simulink model "vehicle_dynamic"  (R2022b)
settings: Solver=VariableStepAuto  StartTime=0.0  StopTime=30  RelTol=1e-3
values from neighbouring files (symbols this model uses):
  vx = 14    [vehicle_lateral_control_LMIs_3states_auto.m]
undefined symbols (not defined in the file or in its folder): K_gain_lin
settings Model: Creator=phatdo  LastModifiedBy=phatdo
settings DataIOCC: ReturnWorkspaceOutputs=off

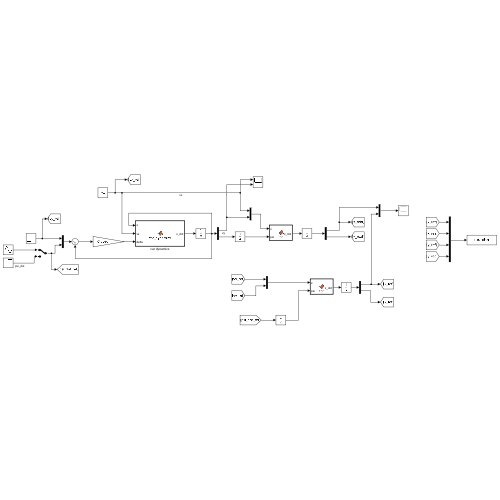
[thumbnail: Simulink's stored preview of the top-level diagram]
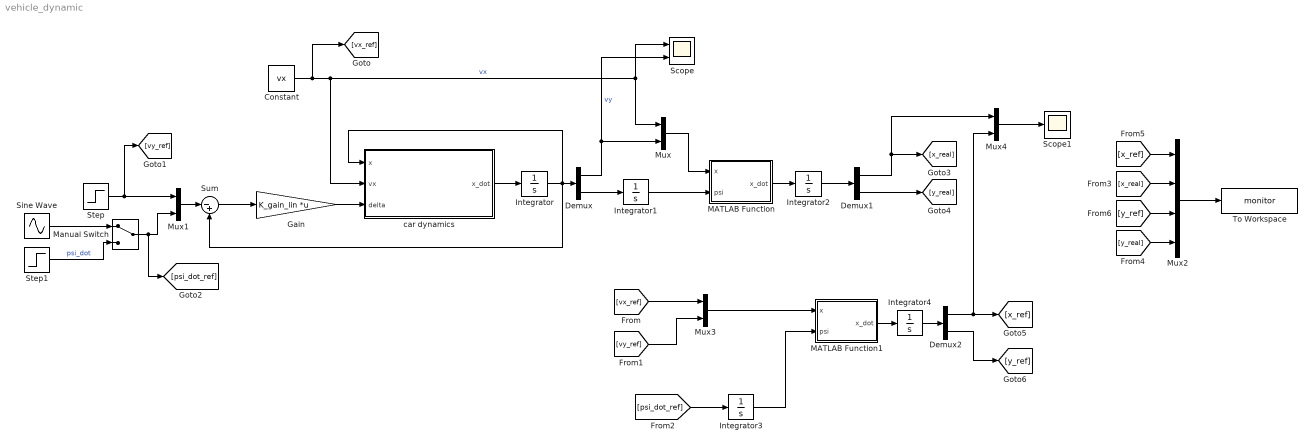
== system vehicle_dynamic ==
  Constant : Constant  Value=vx
  Demux : Demux  Outputs=2
  Demux1 : Demux  Outputs=2
  Demux2 : Demux  Outputs=2
  Gain : Gain  Gain=K_gain_lin  Multiplication=Matrix(K*u) (u vector)
  Integrator{,1..4} (5 alike) : Integrator
  MATLAB Function : MATLAB Function  TreatAsAtomicUnit=on
  MATLAB Function1 : MATLAB Function  TreatAsAtomicUnit=on
  Manual Switch : ManualSwitch
  Mux{,1,3..4} (4 alike) : Mux  Inputs=2
  Mux2 : Mux
  Scope : Scope  NumInputPorts=2
  Scope1 : Scope
  Sine Wave : Sin  SampleTime=0
  Step : Step  Time=0  After=0  SampleTime=0
  Step1 : Step  Time=0  After=0.5  SampleTime=0
  Sum : Sum  Inputs=|-+
  To Workspace : ToWorkspace  VariableName=monitor  SaveFormat=Timeseries  SampleTime=-1
  car dynamics : MATLAB Function  TreatAsAtomicUnit=on
  wires:
  car dynamics/1(x_dot) -> Integrator/1
  Integrator/1 -> car dynamics/1(x), Sum/2, Demux/1
  Constant/1 -> [vx_ref], car dynamics/2(vx), Scope/1, Mux/1  "vx"
  Demux/1 -> Mux/2, Scope/2  "vy"
  Mux/1 -> MATLAB Function/1(x)
  Demux/2 -> Integrator1/1
  Integrator1/1 -> MATLAB Function/2(psi)
  MATLAB Function/1(x_dot) -> Integrator2/1
  Integrator2/1 -> Demux1/1
  Gain/1 -> car dynamics/3(delta)
  Sum/1 -> Gain/1
  Mux1/1 -> Sum/1
  Step/1 -> [vy_ref], Mux1/1
  [psi_dot_ref] -> Integrator3/1
  [vy_ref] -> Mux3/2
  Mux3/1 -> MATLAB Function1/1(x)
  MATLAB Function1/1(x_dot) -> Integrator4/1
  Integrator4/1 -> Demux2/1
  [vx_ref] -> Mux3/1
  Integrator3/1 -> MATLAB Function1/2(psi)
  Demux1/1 -> [x_real], Mux4/1
  Demux1/2 -> [y_real]
  Demux2/1 -> Mux4/2, [x_ref]
  Demux2/2 -> [y_ref]
  [x_ref] -> Mux2/1
  [x_real] -> Mux2/2
  [y_ref] -> Mux2/3
  [y_real] -> Mux2/4
  Mux2/1 -> To Workspace/1
  Mux4/1 -> Scope1/1
  Step1/1 -> Manual Switch/2  "psi_dot"
  Manual Switch/1 -> [psi_dot_ref], Mux1/2
  Sine Wave/1 -> Manual Switch/1

== matlab function vehicle_dynamic/MATLAB Function ==
  data: x input; x_dot output; psi input
function x_dot = fcn(x, psi)

% x = [vx, vy]

x_dot = zeros(2,1);

vx = x(1);
vy = x(2);

x_dot(1) = vx*cos(psi) - vy*sin(psi);
x_dot(2) = vx*sin(psi) + vy*cos(psi);

end

== matlab function vehicle_dynamic/car dynamics ==
  data: x input; vx input; x_dot output; delta input
function x_dot  = car_dynamics(x, vx, delta)

% x_dot = [vy_d, psi_dd]

% x = [vy,psi_d]

x_dot = zeros(2,1);

Cf = 57117;
Cr = 81396;
Iz = 1975;
m = 1621;
lf = 1.15;
lr = 1.38;

vy = x(1);
psi_d = x(2);

x_dot(1) = (-(Cf+Cr)/(m*vx))*vy + ((-lf*Cf+lr*Cr)/(m*vx)-vx)*psi_d + (Cf/m)*delta;

x_dot(2) = ((-lf*Cf+lr*Cr)/(Iz*vx))*vy...
    + (-(lf^2*Cf+lr^2*Cr)/(Iz*vx))*psi_d + (lf*Cf/Iz)*delta;

end

== matlab function vehicle_dynamic/MATLAB Function1 ==
  data: x input; x_dot output; psi input
function x_dot = fcn(x, psi)

% x = [vx, vy]

x_dot = zeros(2,1);

vx = x(1);
vy = x(2);

x_dot(1) = vx*cos(psi) - vy*sin(psi);
x_dot(2) = vx*sin(psi) + vy*cos(psi);

end
